simulink model "svpwm"  (R2021b)
settings: Solver=FixedStepDiscrete  StartTime=0.0  StopTime=0.5  FixedStep=sysStep  RelTol=1e-3
InitFcn:
  | % 华为参数
  | sysStep = 0.5e-6;
  | Udc = 300;
  | PrdPwmCarr = 3125;
  | Ts = 2e-8 * PrdPwmCarr;
  | en7SecMod = true;
  | enModulationUp = true;
  | deadtimeDelay = uint8(5e-6/sysStep); %5us deadtime
  | 
  | %电机参数
  | polepairs = 4;
libraries: spsDiodeLib x6, spsIGBTLib x6, spsVoltageMeasurementLib x3, spsDCVoltageSourceLib x2, spsParallelRLCBranchLib x2, spsGroundLib x1, spsPermanentMagnetSynchronousMachineLib x1, spspowerguiLib x1, simulink x1
settings Model: Creator=zqzq_  LastModifiedBy=zqzq_

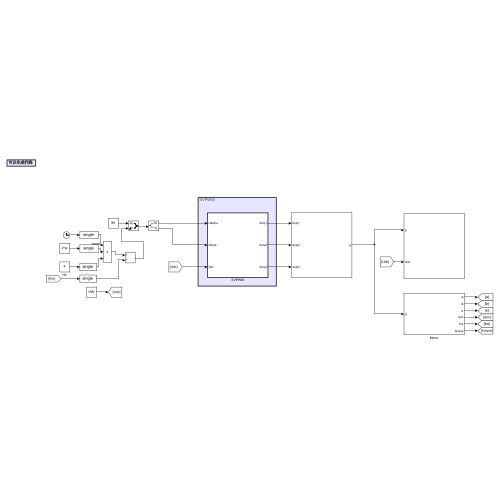
[thumbnail: Simulink's stored preview of the top-level diagram]
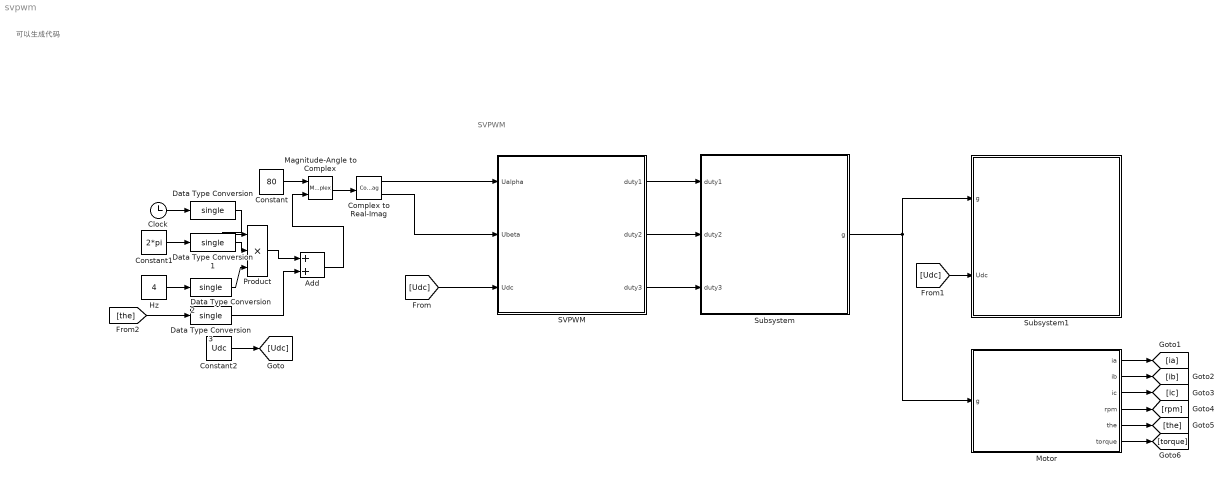
== system svpwm ==
  note: 可以生成代码
  note: SVPWM
  Add : Sum
  Clock : Clock
  Complex to Real-Imag : ComplexToRealImag
  Constant : Constant  Value=80  OutDataTypeStr=Inherit: Inherit via back propagation
  Constant1 : Constant  Value=2*pi  OutDataTypeStr=Inherit: Inherit via back propagation
  Constant2 : Constant  Value=Udc  OutDataTypeStr=Inherit: Inherit via back propagation
  Data Type Conversion{,1..3} (4 alike) : DataTypeConversion  OutDataTypeStr=single
  Hz : Constant  Value=4  OutDataTypeStr=Inherit: Inherit via back propagation
  Magnitude-Angle to Complex : MagnitudeAngleToComplex
  Motor : Subsystem
  Product : Product  Inputs=3
  SVPWM : Subsystem  TreatAsAtomicUnit=on
  Subsystem : Subsystem
  Subsystem1 : Subsystem
  wires:
  Constant2/1 -> [Udc]
  Constant/1 -> Magnitude-Angle to Complex/1
  Complex to Real-Imag/1 -> SVPWM/1(Ualpha)
  Complex to Real-Imag/2 -> SVPWM/2(Ubeta)
  Magnitude-Angle to Complex/1 -> Complex to Real-Imag/1
  Clock/1 -> Data Type Conversion/1
  Constant1/1 -> Data Type Conversion1/1
  Hz/1 -> Data Type Conversion2/1
  Add/1 -> Magnitude-Angle to Complex/2
  Data Type Conversion/1 -> Product/1
  Data Type Conversion1/1 -> Product/2
  Data Type Conversion2/1 -> Product/3
  SVPWM/1(duty1) -> Subsystem/1(duty1)
  SVPWM/2(duty2) -> Subsystem/2(duty2)
  SVPWM/3(duty3) -> Subsystem/3(duty3)
  Subsystem/1(g) -> Motor/1(g), Subsystem1/1(g)
  [Udc] -> SVPWM/3(Udc)
  [Udc] -> Subsystem1/2(Udc)
  Motor/1(ia) -> [ia]
  Motor/2(ib) -> [ib]
  Motor/3(ic) -> [ic]
  Motor/4(rpm) -> [rpm]
  Motor/5(the) -> [the]
  Motor/6(torque) -> [torque]
  [the] -> Data Type Conversion3/1
  Product/1 -> Add/1
  Data Type Conversion3/1 -> Add/2

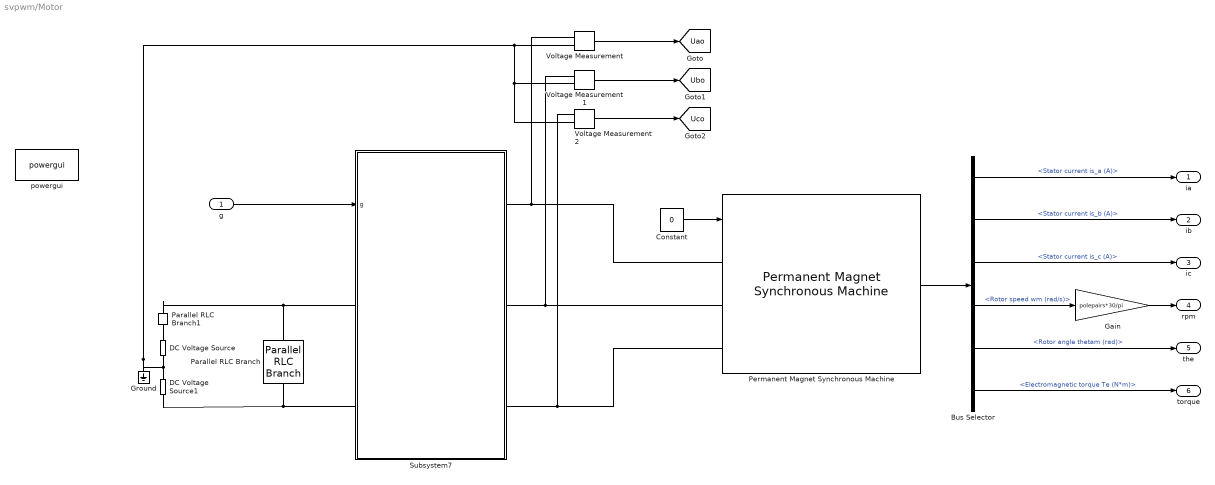
== system svpwm/Motor ==
  g : Inport
  Bus Selector : BusSelector  OutputSignals=Stator current is_a (A),Stator current is_b (A),Stator current is_c (A),Rotor speed wm (rad/s),Rotor angle thetam (rad),Electromagnetic torque Te (N*m)
  Constant : Constant  Value=0  OutDataTypeStr=Inherit: Inherit via back propagation
  DC Voltage Source : spsDCVoltageSourceLib/DC Voltage Source  Amplitude=Udc/2  Measurements=None
  DC Voltage Source1 : spsDCVoltageSourceLib/DC Voltage Source  Amplitude=Udc/2  Measurements=None
  Gain : Gain  Gain=polepairs*30/pi
  Ground : spsGroundLib/Ground  LConnTagsString=a
  Parallel RLC Branch : spsParallelRLCBranchLib/Parallel RLC Branch  LConnTagsString=a  RConnTagsString=__new0  BranchType=C  Resistance=1  Inductance=1e-3  SetiL0=off  InitialCurrent=0  Capacitance=50e-6  Setx0=on  InitialVoltage=Udc  Measurements=None
  Parallel RLC Branch1 : spsParallelRLCBranchLib/Parallel RLC Branch  LConnTagsString=a  RConnTagsString=__new0  BranchType=R  Resistance=0.01  Inductance=1e-3  SetiL0=off  InitialCurrent=0  Capacitance=50e-6  Setx0=on  InitialVoltage=Udc  Measurements=None
  Permanent Magnet Synchronous Machine : spsPermanentMagnetSynchronousMachineLib/Permanent Magnet Synchronous Machine  NbPhases=3  FluxDistribution=Sinusoidal  RotorType=Salient-pole  MechanicalLoad=Speed w  PresetModel="10:  7.71 Nm 560 Vdc 5000 RPM - 10.2 Nm"  ShowDetailedParameters=on  MeasurementBus=off  Resistance=0.18  Inductance=8.5e-3  dqInductances=[0.0007932 0.0008767]  La=0.00097  MachineConstant=Flux linkage established by magnets (V.s)  Flux=0.07145  VoltageCst=51.8384  TorqueCst=0.4287  Flat=120  Mechanical=[0.00062 0.0003035 4 0]  PolePairs=4  InitialConditions=[0,0, 0,0]  InitialConditions5ph=[0 0 0 0 0 0]  RefAngle=90 degrees behind phase A axis (modified Park)  IterativeDiscreteModel=Trapezoidal non iterative  TsBlock=-1  TsPowergui=0
  Subsystem7 : Subsystem
  Voltage Measurement : spsVoltageMeasurementLib/Voltage Measurement  PhasorSimulation=off  OutputType=Complex  PSBequivalent=0
  Voltage Measurement1 : spsVoltageMeasurementLib/Voltage Measurement  PhasorSimulation=off  OutputType=Complex  PSBequivalent=0
  Voltage Measurement2 : spsVoltageMeasurementLib/Voltage Measurement  PhasorSimulation=off  OutputType=Complex  PSBequivalent=0
  powergui : spspowerguiLib/powergui  Priority=1  SimulationMode=Discrete  SampleTime=sysStep  frequency=60  Iterations=50  frequencyindice=0  Pbase=100e6  ErrMax=1e-4  UnitsV=kV  UnitsW=MW  buscounter=0  FunctionMessages=off  echomessages=off  EnableUseOfTLC=off  CurrentSourceSwitches=off  DisableSnubberDevices=off  DisableRonSwitches=off  DisableVfSwitches=off  DisplayEquations=off  AutomaticDiscreteSolvers=off  SolverType=Tustin/Backward Euler (TBE)  Interpol=off  ExternalGateDelay=off  methode=off  Ts=100  x0status=blocks  SPID=on  SwTol=0  HookPort=off  NonlinearTolerance=1e-4  nMaxIteration=100  ContinueOnMaxIteration=off  RestoreLinks=warning  ResistiveCurrentMeasurement=off  Frange=[0:2:500]  Ylog=off  Xlog=on  ShowGrid=off  save=off  variable=ZData  structure=0  ZoomFFT=off  StartTime=0.0  cycles=1  DisplayStyle=1  fundamental=60  FreqAxis=off  MaxFrequency=1000  frequencyindicesteady=1  RmsSteady=1  display=off
  ia : Outport
  ib : Outport  Port=2
  ic : Outport  Port=3
  rpm : Outport  Port=4
  the : Outport  Port=5
  torque : Outport  Port=6
  tag scope: Uao=global, Ubo=global, Uco=global
  wires:
  g/1 -> Subsystem7/1(g)
  Permanent Magnet Synchronous Machine/1 -> Bus Selector/1
  Voltage Measurement/1 -> [Uao]
  Voltage Measurement1/1 -> [Ubo]
  Voltage Measurement2/1 -> [Uco]
  Bus Selector/1 -> ia/1  "<Stator current is_a (A)>"
  Bus Selector/2 -> ib/1  "<Stator current is_b (A)>"
  Bus Selector/3 -> ic/1  "<Stator current is_c (A)>"
  Bus Selector/4 -> Gain/1  "<Rotor speed wm (rad/s)>"
  Bus Selector/5 -> the/1  "<Rotor angle thetam (rad)>"
  Bus Selector/6 -> torque/1  "<Electromagnetic torque Te (N*m)>"
  Gain/1 -> rpm/1
  Constant/1 -> Permanent Magnet Synchronous Machine/1
  connections:
  Subsystem7/RConn2 -- Voltage Measurement1/LConn1 -- Permanent Magnet Synchronous Machine/LConn2
  Parallel RLC Branch/LConn1 -- Parallel RLC Branch1/LConn1 -- Subsystem7/LConn1
  Subsystem7/RConn3 -- Voltage Measurement2/LConn1 -- Permanent Magnet Synchronous Machine/LConn3
  Subsystem7/RConn1 -- Voltage Measurement/LConn1 -- Permanent Magnet Synchronous Machine/LConn1
  Parallel RLC Branch/RConn1 -- DC Voltage Source1/LConn1 -- Subsystem7/LConn2
  Parallel RLC Branch1/RConn1 -- DC Voltage Source/RConn1
  DC Voltage Source/LConn1 -- Voltage Measurement2/LConn2 -- Voltage Measurement1/LConn2 -- Voltage Measurement/LConn2 -- Ground/LConn1 -- DC Voltage Source1/RConn1

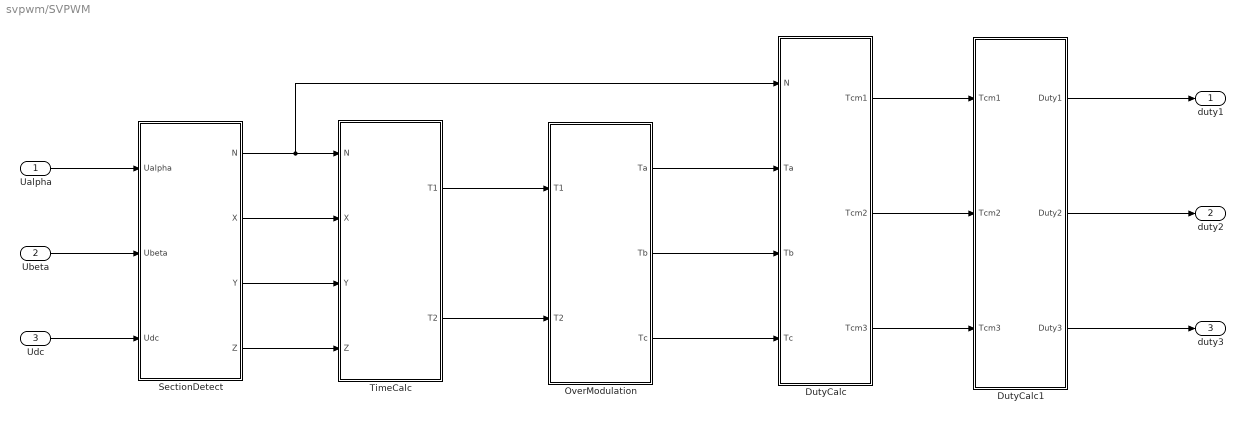
== system svpwm/SVPWM ==
  Ualpha : Inport
  Ubeta : Inport  Port=2
  Udc : Inport  Port=3
  DutyCalc : Subsystem  TreatAsAtomicUnit=on
  DutyCalc1 : Subsystem  TreatAsAtomicUnit=on
  OverModulation : Subsystem  TreatAsAtomicUnit=on
  SectionDetect : Subsystem  TreatAsAtomicUnit=on
  TimeCalc : Subsystem  TreatAsAtomicUnit=on
  duty1 : Outport
  duty2 : Outport  Port=2
  duty3 : Outport  Port=3
  wires:
  Ualpha/1 -> SectionDetect/1(Ualpha)
  Ubeta/1 -> SectionDetect/2(Ubeta)
  Udc/1 -> SectionDetect/3(Udc)
  SectionDetect/1(N) -> DutyCalc/1(N), TimeCalc/1(N)
  SectionDetect/2(X) -> TimeCalc/2(X)
  SectionDetect/3(Y) -> TimeCalc/3(Y)
  SectionDetect/4(Z) -> TimeCalc/4(Z)
  TimeCalc/1(T1) -> OverModulation/1(T1)
  TimeCalc/2(T2) -> OverModulation/2(T2)
  OverModulation/1(Ta) -> DutyCalc/2(Ta)
  OverModulation/2(Tb) -> DutyCalc/3(Tb)
  OverModulation/3(Tc) -> DutyCalc/4(Tc)
  DutyCalc/1(Tcm1) -> DutyCalc1/1(Tcm1)
  DutyCalc/2(Tcm2) -> DutyCalc1/2(Tcm2)
  DutyCalc/3(Tcm3) -> DutyCalc1/3(Tcm3)
  DutyCalc1/1(Duty1) -> duty1/1
  DutyCalc1/3(Duty3) -> duty3/1
  DutyCalc1/2(Duty2) -> duty2/1

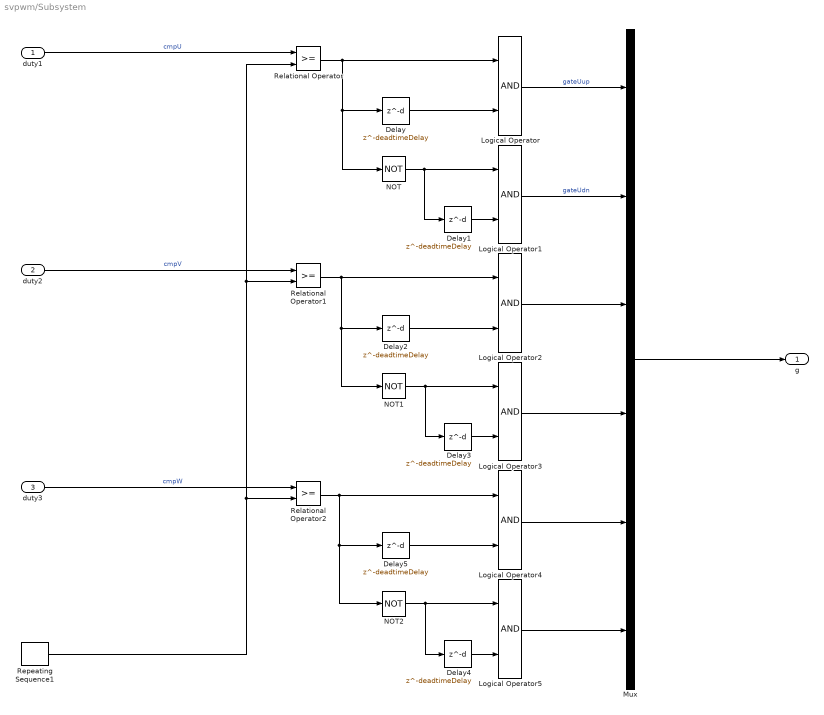
== system svpwm/Subsystem ==
  duty1 : Inport
  duty2 : Inport  Port=2
  duty3 : Inport  Port=3
  Delay{,1..5} (6 alike) : Delay  DelayLength=deadtimeDelay
  Logical Operator{,1..5} (6 alike) : Logic  AllPortsSameDT=off  OutDataTypeStr=boolean
  Mux : Mux  Inputs=6
  NOT : Logic  Operator=NOT  AllPortsSameDT=off  OutDataTypeStr=boolean
  NOT1 : Logic  Operator=NOT  AllPortsSameDT=off  OutDataTypeStr=boolean
  NOT2 : Logic  Operator=NOT  AllPortsSameDT=off  OutDataTypeStr=boolean
  Relational Operator : RelationalOperator  OutDataTypeStr=boolean  RndMeth=Simplest
  Relational Operator1 : RelationalOperator  OutDataTypeStr=boolean  RndMeth=Simplest
  Relational Operator2 : RelationalOperator  OutDataTypeStr=boolean  RndMeth=Simplest
  Repeating Sequence1 : simulink/Sources/Repeating Sequence  rep_seq_t=[0 2e-8*PrdPwmCarr 4e-8*PrdPwmCarr]  rep_seq_y=[0.001 0.999 0.001]
  g : Outport
  wires:
  duty1/1 -> Relational Operator/1  "cmpU"
  duty2/1 -> Relational Operator1/1  "cmpV"
  Mux/1 -> g/1
  Logical Operator/1 -> Mux/1  "gateUup"
  Logical Operator1/1 -> Mux/2  "gateUdn"
  Logical Operator2/1 -> Mux/3
  Logical Operator3/1 -> Mux/4
  Logical Operator4/1 -> Mux/5
  Logical Operator5/1 -> Mux/6
  Repeating Sequence1/1 -> Relational Operator2/2, Relational Operator/2, Relational Operator1/2
  Relational Operator/1 -> Delay/1, NOT/1, Logical Operator/1
  NOT/1 -> Delay1/1, Logical Operator1/1
  duty3/1 -> Relational Operator2/1  "cmpW"
  NOT1/1 -> Delay3/1, Logical Operator3/1
  Relational Operator1/1 -> Delay2/1, NOT1/1, Logical Operator2/1
  NOT2/1 -> Delay4/1, Logical Operator5/1
  Delay/1 -> Logical Operator/2
  Delay1/1 -> Logical Operator1/2
  Delay2/1 -> Logical Operator2/2
  Delay3/1 -> Logical Operator3/2
  Delay4/1 -> Logical Operator5/2
  Relational Operator2/1 -> Delay5/1, NOT2/1, Logical Operator4/1
  Delay5/1 -> Logical Operator4/2

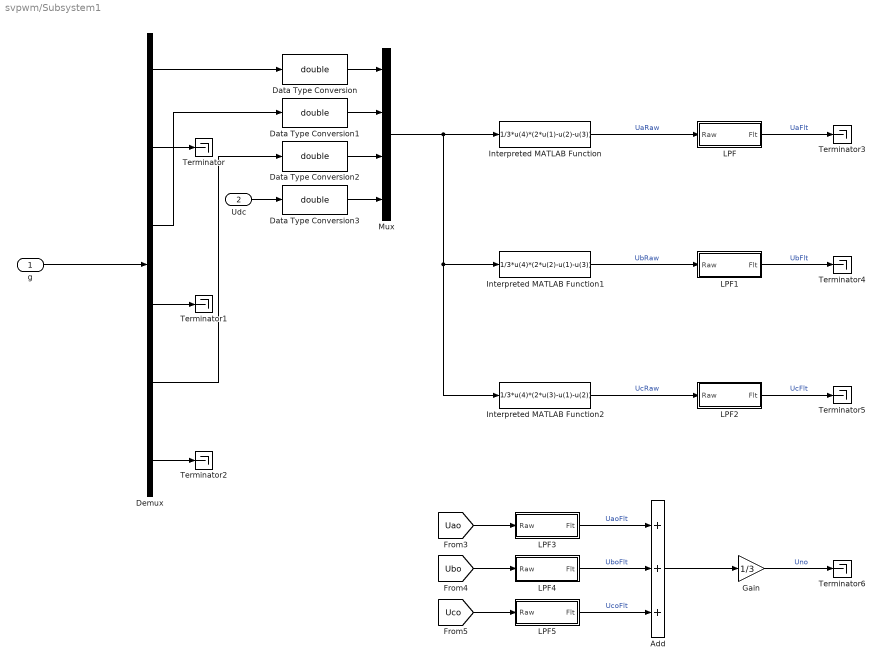
== system svpwm/Subsystem1 ==
  g : Inport
  Udc : Inport  Port=2  OutDataTypeStr=single
  Add : Sum  Inputs=+++
  Data Type Conversion{,1..3} (4 alike) : DataTypeConversion  OutDataTypeStr=double
  Demux : Demux  Outputs=6
  Gain : Gain  Gain=1/3
  Interpreted MATLAB Function : MATLABFcn  MATLABFcn=1/3*u(4)*(2*u(1)-u(2)-u(3))  OutputSignalType=real
  Interpreted MATLAB Function1 : MATLABFcn  MATLABFcn=1/3*u(4)*(2*u(2)-u(1)-u(3))  OutputSignalType=real
  Interpreted MATLAB Function2 : MATLABFcn  MATLABFcn=1/3*u(4)*(2*u(3)-u(1)-u(2))  OutputSignalType=real
  LPF : Subsystem  TreatAsAtomicUnit=on
  LPF1 : Subsystem  TreatAsAtomicUnit=on
  LPF2 : Subsystem  TreatAsAtomicUnit=on
  LPF3 : Subsystem  TreatAsAtomicUnit=on
  LPF4 : Subsystem  TreatAsAtomicUnit=on
  LPF5 : Subsystem  TreatAsAtomicUnit=on
  Mux : Mux
  Terminator{,1..6} (7 alike) : Terminator
  wires:
  g/1 -> Demux/1
  Demux/2 -> Terminator/1
  Demux/4 -> Terminator1/1
  Demux/6 -> Terminator2/1
  Demux/1 -> Data Type Conversion/1
  Demux/3 -> Data Type Conversion1/1
  Demux/5 -> Data Type Conversion2/1
  Udc/1 -> Data Type Conversion3/1
  Interpreted MATLAB Function/1 -> LPF/1(Raw)  "UaRaw"
  Interpreted MATLAB Function1/1 -> LPF1/1(Raw)  "UbRaw"
  Interpreted MATLAB Function2/1 -> LPF2/1(Raw)  "UcRaw"
  Mux/1 -> Interpreted MATLAB Function2/1, Interpreted MATLAB Function1/1, Interpreted MATLAB Function/1
  Data Type Conversion/1 -> Mux/1
  Data Type Conversion1/1 -> Mux/2
  Data Type Conversion2/1 -> Mux/3
  Data Type Conversion3/1 -> Mux/4
  LPF/1(Flt) -> Terminator3/1  "UaFlt"
  LPF1/1(Flt) -> Terminator4/1  "UbFlt"
  LPF2/1(Flt) -> Terminator5/1  "UcFlt"
  Add/1 -> Gain/1
  Gain/1 -> Terminator6/1  "Uno"
  [Uao] -> LPF3/1(Raw)
  [Ubo] -> LPF4/1(Raw)
  [Uco] -> LPF5/1(Raw)
  LPF3/1(Flt) -> Add/1  "UaoFlt"
  LPF4/1(Flt) -> Add/2  "UboFlt"
  LPF5/1(Flt) -> Add/3  "UcoFlt"

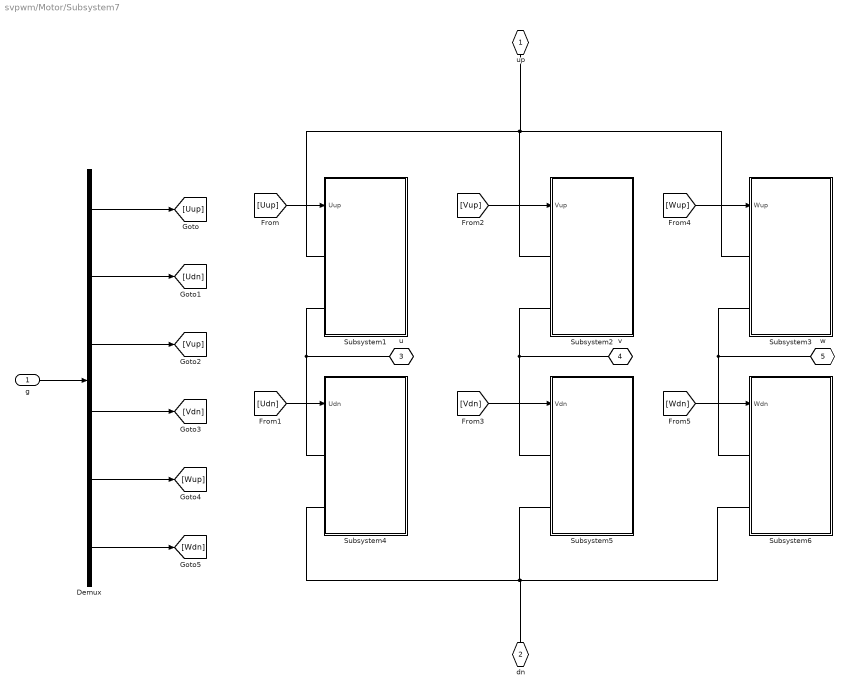
== system svpwm/Motor/Subsystem7 ==
  g : Inport
  Demux : Demux  Outputs=6
  Subsystem1 : Subsystem
  Subsystem2 : Subsystem
  Subsystem3 : Subsystem
  Subsystem4 : Subsystem
  Subsystem5 : Subsystem
  Subsystem6 : Subsystem
  up : PMIOPort  Side=Left
  dn : PMIOPort  Port=2  Side=Left
  u : PMIOPort  Port=3  Side=Right
  v : PMIOPort  Port=4  Side=Right
  w : PMIOPort  Port=5  Side=Right
  wires:
  g/1 -> Demux/1
  Demux/1 -> [Uup]
  Demux/2 -> [Udn]
  Demux/3 -> [Vup]
  Demux/4 -> [Vdn]
  Demux/5 -> [Wup]
  Demux/6 -> [Wdn]
  [Uup] -> Subsystem1/1(Uup)
  [Udn] -> Subsystem4/1(Udn)
  [Vup] -> Subsystem2/1(Vup)
  [Vdn] -> Subsystem5/1(Vdn)
  [Wup] -> Subsystem3/1(Wup)
  [Wdn] -> Subsystem6/1(Wdn)
  connections:
  Subsystem3/LConn2 -- w/RConn1 -- Subsystem6/LConn1
  Subsystem4/LConn2 -- Subsystem6/LConn2 -- dn/RConn1 -- Subsystem5/LConn2
  Subsystem1/LConn1 -- Subsystem3/LConn1 -- up/RConn1 -- Subsystem2/LConn1
  Subsystem2/LConn2 -- v/RConn1 -- Subsystem5/LConn1
  Subsystem1/LConn2 -- u/RConn1 -- Subsystem4/LConn1

== system svpwm/SVPWM/DutyCalc ==
  N : Inport
  Ta : Inport  Port=2
  Tb : Inport  Port=3
  Tc : Inport  Port=4
  Multiport Switch : MultiPortSwitch  Inputs=6
  Multiport Switch1 : MultiPortSwitch  Inputs=6
  Multiport Switch2 : MultiPortSwitch  Inputs=6
  Tcm1 : Outport
  Tcm2 : Outport  Port=2
  Tcm3 : Outport  Port=3
  wires:
  Multiport Switch2/1 -> Tcm3/1
  Multiport Switch1/1 -> Tcm2/1
  Multiport Switch/1 -> Tcm1/1
  Ta/1 -> Multiport Switch2/7, Multiport Switch2/5, Multiport Switch1/6, Multiport Switch1/2, Multiport Switch/3, Multiport Switch/4
  Tb/1 -> Multiport Switch2/6, Multiport Switch2/3, Multiport Switch1/5, Multiport Switch1/4, Multiport Switch/7, Multiport Switch/2
  N/1 -> Multiport Switch2/1, Multiport Switch1/1, Multiport Switch/1
  Tc/1 -> Multiport Switch2/4, Multiport Switch/6, Multiport Switch/5, Multiport Switch1/3, Multiport Switch1/7, Multiport Switch2/2

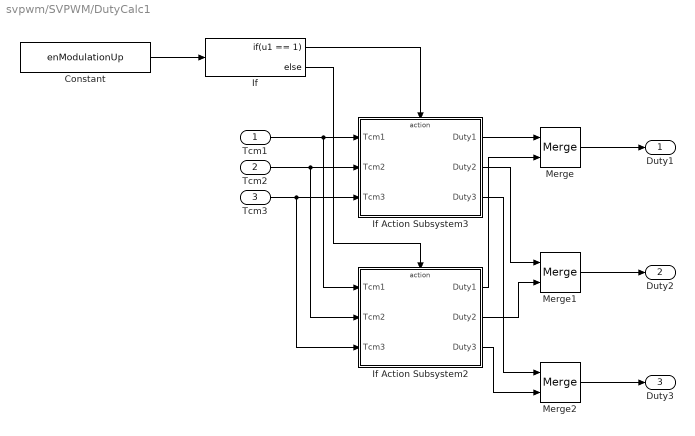
== system svpwm/SVPWM/DutyCalc1 ==
  Tcm1 : Inport
  Tcm2 : Inport  Port=2
  Tcm3 : Inport  Port=3
  Constant : Constant  Value=enModulationUp
  If : If  IfExpression=u1 == 1
  If Action Subsystem2 : Subsystem  TreatAsAtomicUnit=on
  If Action Subsystem3 : Subsystem  TreatAsAtomicUnit=on
  Merge : Merge
  Merge1 : Merge
  Merge2 : Merge
  Duty1 : Outport
  Duty2 : Outport  Port=2
  Duty3 : Outport  Port=3
  wires:
  Constant/1 -> If/1
  If/1 -> If Action Subsystem3/Action
  Tcm1/1 -> If Action Subsystem2/1(Tcm1), If Action Subsystem3/1(Tcm1)
  Tcm2/1 -> If Action Subsystem2/2(Tcm2), If Action Subsystem3/2(Tcm2)
  Tcm3/1 -> If Action Subsystem2/3(Tcm3), If Action Subsystem3/3(Tcm3)
  If Action Subsystem3/1(Duty1) -> Merge/1
  If/2 -> If Action Subsystem2/Action
  Merge/1 -> Duty1/1
  Merge1/1 -> Duty2/1
  If Action Subsystem3/2(Duty2) -> Merge1/1
  Merge2/1 -> Duty3/1
  If Action Subsystem3/3(Duty3) -> Merge2/1
  If Action Subsystem2/3(Duty3) -> Merge2/2
  If Action Subsystem2/2(Duty2) -> Merge1/2
  If Action Subsystem2/1(Duty1) -> Merge/2

== system svpwm/SVPWM/OverModulation ==
  T1 : Inport
  T2 : Inport  Port=2
  OverModulationCalc : Subsystem  TreatAsAtomicUnit=on
  TabcCalc : Subsystem  TreatAsAtomicUnit=on
  Ta : Outport
  Tb : Outport  Port=2
  Tc : Outport  Port=3
  wires:
  T2/1 -> OverModulationCalc/2(T2)
  T1/1 -> OverModulationCalc/1(T1)
  OverModulationCalc/2(T2_) -> TabcCalc/2(T2_)
  TabcCalc/1(Ta) -> Ta/1
  TabcCalc/2(Tb) -> Tb/1
  TabcCalc/3(Tc) -> Tc/1
  OverModulationCalc/1(T1_) -> TabcCalc/1(T1_)

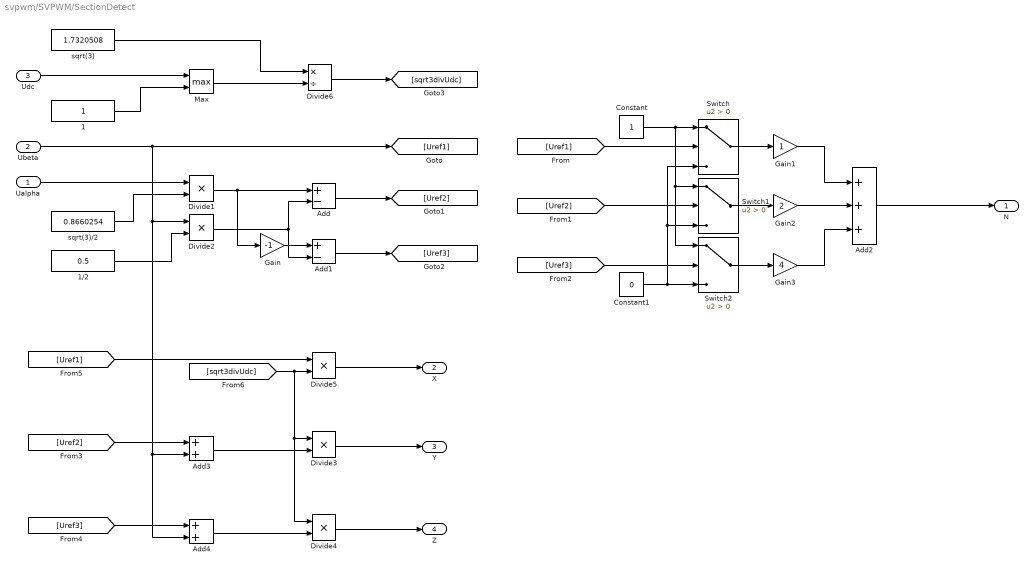
== system svpwm/SVPWM/SectionDetect ==
  Ualpha : Inport
  Ubeta : Inport  Port=2
  Udc : Inport  Port=3
  1 : Constant  OutDataTypeStr=single
  1/2 : Constant  Value=0.5  OutDataTypeStr=single
  Add : Sum  Inputs=+-
  Add1 : Sum  Inputs=+-
  Add2 : Sum  Inputs=+++
  Add3 : Sum
  Add4 : Sum
  Constant : Constant  OutDataTypeStr=uint8
  Constant1 : Constant  Value=0  OutDataTypeStr=uint8
  Divide{1..5} (5 alike) : Product  Inputs=**
  Divide6 : Product  Inputs=*/
  Gain : Gain  Gain=-1
  Gain1 : Gain
  Gain2 : Gain  Gain=2
  Gain3 : Gain  Gain=4
  Max : MinMax  Function=max  Inputs=2
  Switch : Switch  Criteria=u2 > Threshold
  Switch1 : Switch  Criteria=u2 > Threshold
  Switch2 : Switch  Criteria=u2 > Threshold
  sqrt(3) : Constant  Value=1.7320508  OutDataTypeStr=single
  sqrt(3)/2 : Constant  Value=0.8660254  OutDataTypeStr=single
  N : Outport
  X : Outport  Port=2
  Y : Outport  Port=3
  Z : Outport  Port=4
  wires:
  Ubeta/1 -> [Uref1], Add4/2, Add3/2, Divide2/1
  Ualpha/1 -> Divide1/1
  Divide1/1 -> Gain/1, Add/1
  sqrt(3)/2/1 -> Divide1/2
  1/2/1 -> Divide2/2
  Add/1 -> [Uref2]
  Divide2/1 -> Add1/2, Add/2
  Add1/1 -> [Uref3]
  Gain/1 -> Add1/1
  [Uref1] -> Switch/2
  Constant/1 -> Switch2/1, Switch1/1, Switch/1
  Constant1/1 -> Switch/3, Switch1/3, Switch2/3
  Switch/1 -> Gain1/1
  [Uref2] -> Switch1/2
  Switch1/1 -> Gain2/1
  Switch2/1 -> Gain3/1
  [Uref3] -> Switch2/2
  Gain2/1 -> Add2/2
  Gain1/1 -> Add2/1
  Gain3/1 -> Add2/3
  Add2/1 -> N/1
  [Uref2] -> Add3/1
  [Uref3] -> Add4/1
  Add3/1 -> Divide3/2
  Add4/1 -> Divide4/2
  [Uref1] -> Divide5/1
  Udc/1 -> Max/1
  1/1 -> Max/2
  Max/1 -> Divide6/2
  sqrt(3)/1 -> Divide6/1
  Divide6/1 -> [sqrt3divUdc]
  [sqrt3divUdc] -> Divide3/1, Divide4/1, Divide5/2
  Divide5/1 -> X/1
  Divide3/1 -> Y/1
  Divide4/1 -> Z/1

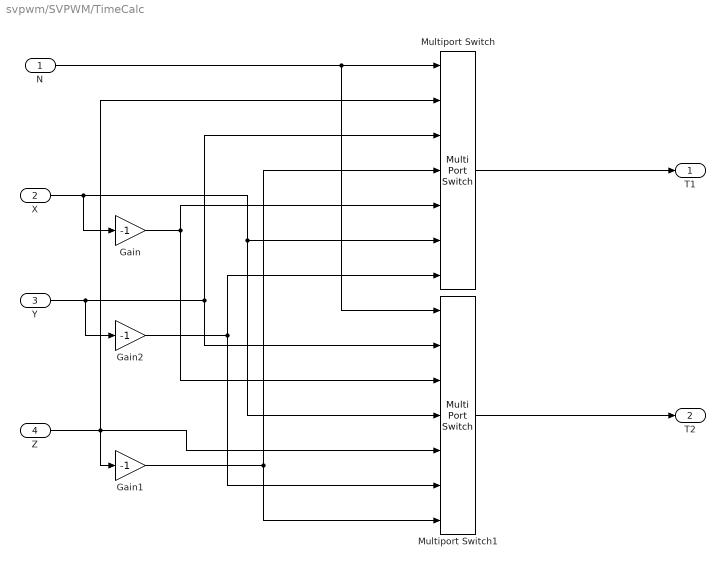
== system svpwm/SVPWM/TimeCalc ==
  N : Inport
  X : Inport  Port=2
  Y : Inport  Port=3
  Z : Inport  Port=4
  Gain : Gain  Gain=-1
  Gain1 : Gain  Gain=-1
  Gain2 : Gain  Gain=-1
  Multiport Switch : MultiPortSwitch  Inputs=6
  Multiport Switch1 : MultiPortSwitch  Inputs=6
  T1 : Outport
  T2 : Outport  Port=2
  wires:
  N/1 -> Multiport Switch1/1, Multiport Switch/1
  Z/1 -> Multiport Switch1/5, Gain1/1, Multiport Switch/2
  X/1 -> Multiport Switch1/4, Multiport Switch/6, Gain/1
  Gain/1 -> Multiport Switch/5, Multiport Switch1/3
  Y/1 -> Multiport Switch/3, Multiport Switch1/2, Gain2/1
  Gain2/1 -> Multiport Switch1/6, Multiport Switch/7
  Gain1/1 -> Multiport Switch/4, Multiport Switch1/7
  Multiport Switch/1 -> T1/1
  Multiport Switch1/1 -> T2/1

== system svpwm/Subsystem1/LPF ==
  Raw : Inport
  Add : Sum
  Add1 : Sum  Inputs=+-
  Constant : Constant  Value=0.001  OutDataTypeStr=Inherit: Inherit via back propagation
  Constant1 : Constant  OutDataTypeStr=Inherit: Inherit via back propagation
  Delay : Delay  DelayLength=1
  Product : Product
  Product1 : Product
  Flt : Outport
  wires:
  Raw/1 -> Product1/1
  Add/1 -> Delay/1, Flt/1
  Delay/1 -> Product/2
  Product/1 -> Add/2
  Constant/1 -> Add1/2, Product1/2
  Product1/1 -> Add/1
  Add1/1 -> Product/1
  Constant1/1 -> Add1/1

== system svpwm/Subsystem1/LPF1 ==
  Raw : Inport
  Add : Sum
  Add1 : Sum  Inputs=+-
  Constant : Constant  Value=0.001  OutDataTypeStr=Inherit: Inherit via back propagation
  Constant1 : Constant  OutDataTypeStr=Inherit: Inherit via back propagation
  Delay : Delay  DelayLength=1
  Product : Product
  Product1 : Product
  Flt : Outport
  wires:
  Constant1/1 -> Add1/1
  Add1/1 -> Product/1
  Product1/1 -> Add/1
  Constant/1 -> Product1/2, Add1/2
  Product/1 -> Add/2
  Delay/1 -> Product/2
  Add/1 -> Flt/1, Delay/1
  Raw/1 -> Product1/1

== system svpwm/Subsystem1/LPF2 ==
  Raw : Inport
  Add : Sum
  Add1 : Sum  Inputs=+-
  Constant : Constant  Value=0.001  OutDataTypeStr=Inherit: Inherit via back propagation
  Constant1 : Constant  OutDataTypeStr=Inherit: Inherit via back propagation
  Delay : Delay  DelayLength=1
  Product : Product
  Product1 : Product
  Flt : Outport
  wires:
  Raw/1 -> Product1/1
  Add/1 -> Delay/1, Flt/1
  Delay/1 -> Product/2
  Product/1 -> Add/2
  Constant/1 -> Add1/2, Product1/2
  Product1/1 -> Add/1
  Add1/1 -> Product/1
  Constant1/1 -> Add1/1

== system svpwm/Subsystem1/LPF3 ==
  Raw : Inport
  Add : Sum
  Add1 : Sum  Inputs=+-
  Constant : Constant  Value=0.0004  OutDataTypeStr=Inherit: Inherit via back propagation
  Constant1 : Constant  OutDataTypeStr=Inherit: Inherit via back propagation
  Delay : Delay  DelayLength=1
  Product : Product
  Product1 : Product
  Flt : Outport
  wires:
  Constant1/1 -> Add1/1
  Add1/1 -> Product/1
  Product1/1 -> Add/1
  Constant/1 -> Product1/2, Add1/2
  Product/1 -> Add/2
  Delay/1 -> Product/2
  Add/1 -> Flt/1, Delay/1
  Raw/1 -> Product1/1

== system svpwm/Subsystem1/LPF4 ==
  Raw : Inport
  Add : Sum
  Add1 : Sum  Inputs=+-
  Constant : Constant  Value=0.0004  OutDataTypeStr=Inherit: Inherit via back propagation
  Constant1 : Constant  OutDataTypeStr=Inherit: Inherit via back propagation
  Delay : Delay  DelayLength=1
  Product : Product
  Product1 : Product
  Flt : Outport
  wires:
  Raw/1 -> Product1/1
  Add/1 -> Delay/1, Flt/1
  Delay/1 -> Product/2
  Product/1 -> Add/2
  Constant/1 -> Add1/2, Product1/2
  Product1/1 -> Add/1
  Add1/1 -> Product/1
  Constant1/1 -> Add1/1

== system svpwm/Subsystem1/LPF5 ==
  Raw : Inport
  Add : Sum
  Add1 : Sum  Inputs=+-
  Constant : Constant  Value=0.0004  OutDataTypeStr=Inherit: Inherit via back propagation
  Constant1 : Constant  OutDataTypeStr=Inherit: Inherit via back propagation
  Delay : Delay  DelayLength=1
  Product : Product
  Product1 : Product
  Flt : Outport
  wires:
  Constant1/1 -> Add1/1
  Add1/1 -> Product/1
  Product1/1 -> Add/1
  Constant/1 -> Product1/2, Add1/2
  Product/1 -> Add/2
  Delay/1 -> Product/2
  Add/1 -> Flt/1, Delay/1
  Raw/1 -> Product1/1

== system svpwm/Motor/Subsystem7/Subsystem1 ==
  Uup : Inport
  Diode : spsDiodeLib/Diode  Ron=0.001  Lon=0  Vf=0.8  IC=0  UseSnubber=0  Rs=500  Cs=250e-9  Measurements=on
  IGBT : spsIGBTLib/IGBT  Ron=0.001  Lon=0  Vf=1  Tf=1e-6  Tt=2e-6  IC=0  Rs=1e5  Cs=inf  Measurements=on
  Terminator : Terminator
  Terminator1 : Terminator
  up : PMIOPort  Side=Left
  dn : PMIOPort  Port=2  Side=Left
  wires:
  Diode/1 -> Terminator/1
  IGBT/1 -> Terminator1/1
  Uup/1 -> IGBT/1
  connections:
  Diode/LConn1 -- dn/RConn1 -- IGBT/RConn1
  Diode/RConn1 -- IGBT/LConn1 -- up/RConn1

== system svpwm/Motor/Subsystem7/Subsystem2 ==
  Vup : Inport
  Diode : spsDiodeLib/Diode  Ron=0.001  Lon=0  Vf=0.8  IC=0  UseSnubber=0  Rs=500  Cs=250e-9  Measurements=on
  IGBT : spsIGBTLib/IGBT  Ron=0.001  Lon=0  Vf=1  Tf=1e-6  Tt=2e-6  IC=0  Rs=1e5  Cs=inf  Measurements=on
  Terminator : Terminator
  Terminator1 : Terminator
  up : PMIOPort  Side=Left
  dn : PMIOPort  Port=2  Side=Left
  wires:
  Vup/1 -> IGBT/1
  IGBT/1 -> Terminator1/1
  Diode/1 -> Terminator/1
  connections:
  IGBT/LConn1 -- Diode/RConn1 -- up/RConn1
  dn/RConn1 -- Diode/LConn1 -- IGBT/RConn1

== system svpwm/Motor/Subsystem7/Subsystem3 ==
  Wup : Inport
  Diode : spsDiodeLib/Diode  Ron=0.001  Lon=0  Vf=0.8  IC=0  UseSnubber=0  Rs=500  Cs=250e-9  Measurements=on
  IGBT : spsIGBTLib/IGBT  Ron=0.001  Lon=0  Vf=1  Tf=1e-6  Tt=2e-6  IC=0  Rs=1e5  Cs=inf  Measurements=on
  Terminator : Terminator
  Terminator1 : Terminator
  up : PMIOPort  Side=Left
  dn : PMIOPort  Port=2  Side=Left
  wires:
  Diode/1 -> Terminator/1
  IGBT/1 -> Terminator1/1
  Wup/1 -> IGBT/1
  connections:
  IGBT/RConn1 -- Diode/LConn1 -- dn/RConn1
  up/RConn1 -- Diode/RConn1 -- IGBT/LConn1

== system svpwm/Motor/Subsystem7/Subsystem4 ==
  Udn : Inport
  Diode : spsDiodeLib/Diode  Ron=0.001  Lon=0  Vf=0.8  IC=0  UseSnubber=0  Rs=500  Cs=250e-9  Measurements=on
  IGBT : spsIGBTLib/IGBT  Ron=0.001  Lon=0  Vf=1  Tf=1e-6  Tt=2e-6  IC=0  Rs=1e5  Cs=inf  Measurements=on
  Terminator : Terminator
  Terminator1 : Terminator
  up : PMIOPort  Side=Left
  dn : PMIOPort  Port=2  Side=Left
  wires:
  Udn/1 -> IGBT/1
  IGBT/1 -> Terminator1/1
  Diode/1 -> Terminator/1
  connections:
  IGBT/LConn1 -- Diode/RConn1 -- up/RConn1
  dn/RConn1 -- Diode/LConn1 -- IGBT/RConn1

== system svpwm/Motor/Subsystem7/Subsystem5 ==
  Vdn : Inport
  Diode : spsDiodeLib/Diode  Ron=0.001  Lon=0  Vf=0.8  IC=0  UseSnubber=0  Rs=500  Cs=250e-9  Measurements=on
  IGBT : spsIGBTLib/IGBT  Ron=0.001  Lon=0  Vf=1  Tf=1e-6  Tt=2e-6  IC=0  Rs=1e5  Cs=inf  Measurements=on
  Terminator : Terminator
  Terminator1 : Terminator
  up : PMIOPort  Side=Left
  dn : PMIOPort  Port=2  Side=Left
  wires:
  Diode/1 -> Terminator/1
  IGBT/1 -> Terminator1/1
  Vdn/1 -> IGBT/1
  connections:
  IGBT/RConn1 -- Diode/LConn1 -- dn/RConn1
  up/RConn1 -- Diode/RConn1 -- IGBT/LConn1

== system svpwm/Motor/Subsystem7/Subsystem6 ==
  Wdn : Inport
  Diode : spsDiodeLib/Diode  Ron=0.001  Lon=0  Vf=0.8  IC=0  UseSnubber=0  Rs=500  Cs=250e-9  Measurements=on
  IGBT : spsIGBTLib/IGBT  Ron=0.001  Lon=0  Vf=1  Tf=1e-6  Tt=2e-6  IC=0  Rs=1e5  Cs=inf  Measurements=on
  Terminator : Terminator
  Terminator1 : Terminator
  up : PMIOPort  Side=Left
  dn : PMIOPort  Port=2  Side=Left
  wires:
  Wdn/1 -> IGBT/1
  IGBT/1 -> Terminator1/1
  Diode/1 -> Terminator/1
  connections:
  IGBT/LConn1 -- Diode/RConn1 -- up/RConn1
  dn/RConn1 -- Diode/LConn1 -- IGBT/RConn1

== system svpwm/SVPWM/DutyCalc1/If Action Subsystem2 ==
  Tcm1 : Inport
  Tcm2 : Inport  Port=2
  Tcm3 : Inport  Port=3
  Action Port : ActionPort  ActionPortLabel=else
  Duty1 : Outport
  Duty2 : Outport  Port=2
  Duty3 : Outport  Port=3
  wires:
  Tcm1/1 -> Duty1/1
  Tcm2/1 -> Duty2/1
  Tcm3/1 -> Duty3/1

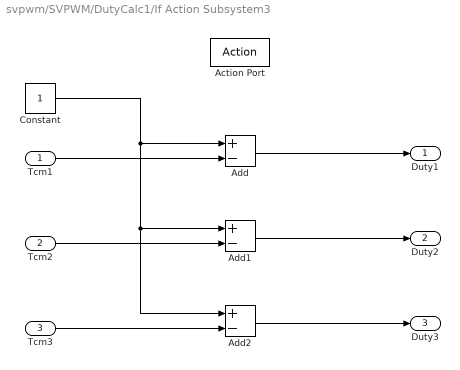
== system svpwm/SVPWM/DutyCalc1/If Action Subsystem3 ==
  Tcm1 : Inport
  Tcm2 : Inport  Port=2
  Tcm3 : Inport  Port=3
  Action Port : ActionPort  ActionPortLabel=if(u1 == 1)
  Add : Sum  Inputs=+-
  Add1 : Sum  Inputs=+-
  Add2 : Sum  Inputs=+-
  Constant : Constant  OutDataTypeStr=Inherit: Inherit via back propagation
  Duty1 : Outport
  Duty2 : Outport  Port=2
  Duty3 : Outport  Port=3
  wires:
  Add2/1 -> Duty3/1
  Add1/1 -> Duty2/1
  Add/1 -> Duty1/1
  Tcm3/1 -> Add2/2
  Tcm2/1 -> Add1/2
  Tcm1/1 -> Add/2
  Constant/1 -> Add/1, Add1/1, Add2/1

== system svpwm/SVPWM/OverModulation/OverModulationCalc ==
  T1 : Inport
  T2 : Inport  Port=2
  Add : Sum
  If : If  IfExpression=u1 > 1
  If Action Subsystem : Subsystem  TreatAsAtomicUnit=on
  If Action Subsystem1 : Subsystem  TreatAsAtomicUnit=on
  Merge : Merge
  Merge1 : Merge
  T1_ : Outport
  T2_ : Outport  Port=2
  wires:
  Merge/1 -> T1_/1
  If/1 -> If Action Subsystem/Action
  If/2 -> If Action Subsystem1/Action
  If Action Subsystem/1(T1_) -> Merge/1
  If Action Subsystem1/1(T1_) -> Merge/2
  If Action Subsystem1/2(T2_) -> Merge1/2
  Merge1/1 -> T2_/1
  If Action Subsystem/2(T2_) -> Merge1/1
  T2/1 -> If Action Subsystem1/2(T2), If Action Subsystem/2(T2), Add/2
  T1/1 -> If Action Subsystem/1(T1), If Action Subsystem1/1(T1), Add/1
  Add/1 -> If Action Subsystem/3(Sum), If/1

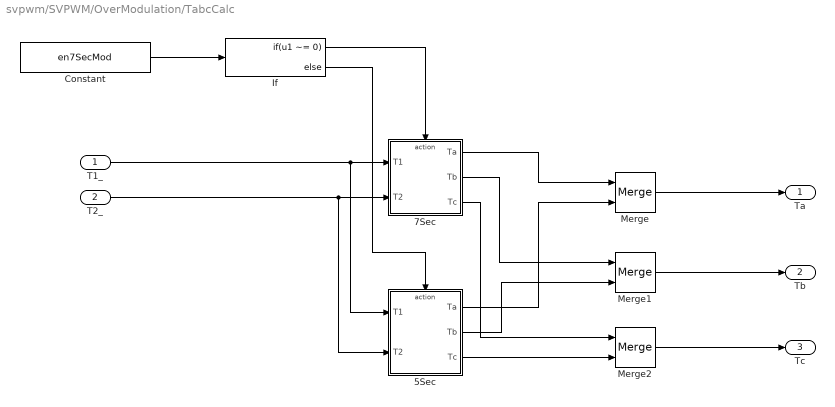
== system svpwm/SVPWM/OverModulation/TabcCalc ==
  T1_ : Inport
  T2_ : Inport  Port=2
  5Sec : Subsystem  TreatAsAtomicUnit=on
  7Sec : Subsystem  TreatAsAtomicUnit=on
  Constant : Constant  Value=en7SecMod
  If : If  IfExpression=u1 ~= 0
  Merge : Merge
  Merge1 : Merge
  Merge2 : Merge
  Ta : Outport
  Tb : Outport  Port=2
  Tc : Outport  Port=3
  wires:
  Constant/1 -> If/1
  If/1 -> 7Sec/Action
  If/2 -> 5Sec/Action
  T1_/1 -> 5Sec/1(T1), 7Sec/1(T1)
  T2_/1 -> 5Sec/2(T2), 7Sec/2(T2)
  Merge/1 -> Ta/1
  7Sec/1(Ta) -> Merge/1
  5Sec/1(Ta) -> Merge/2
  Merge1/1 -> Tb/1
  Merge2/1 -> Tc/1
  7Sec/2(Tb) -> Merge1/1
  5Sec/2(Tb) -> Merge1/2
  7Sec/3(Tc) -> Merge2/1
  5Sec/3(Tc) -> Merge2/2

== system svpwm/SVPWM/OverModulation/OverModulationCalc/If Action Subsystem ==
  T1 : Inport
  T2 : Inport  Port=2
  Sum : Inport  Port=3
  Action Port : ActionPort  ActionPortLabel=if(u1 > 1)
  Divide : Product  Inputs=*/
  Divide1 : Product  Inputs=*/
  T1_ : Outport
  T2_ : Outport  Port=2
  wires:
  T1/1 -> Divide/1
  T2/1 -> Divide1/1
  Sum/1 -> Divide/2, Divide1/2
  Divide/1 -> T1_/1
  Divide1/1 -> T2_/1

== system svpwm/SVPWM/OverModulation/OverModulationCalc/If Action Subsystem1 ==
  T1 : Inport
  T2 : Inport  Port=2
  Action Port : ActionPort  ActionPortLabel=else
  T1_ : Outport
  T2_ : Outport  Port=2
  wires:
  T1/1 -> T1_/1
  T2/1 -> T2_/1

== system svpwm/SVPWM/OverModulation/TabcCalc/5Sec ==
  note: 零矢量选择全部为U7(1,1,1)
  T1 : Inport
  T2 : Inport  Port=2
  Action Port : ActionPort  ActionPortLabel=else
  Add2 : Sum
  Constant : Constant  Value=0  OutDataTypeStr=single
  Ta : Outport
  Tb : Outport  Port=2
  Tc : Outport  Port=3
  wires:
  Add2/1 -> Tc/1
  T2/1 -> Tb/1, Add2/1
  T1/1 -> Add2/2
  Constant/1 -> Ta/1

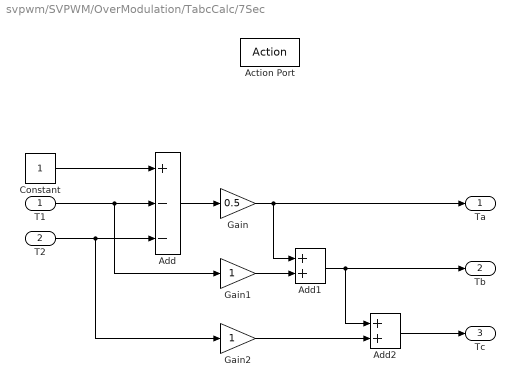
== system svpwm/SVPWM/OverModulation/TabcCalc/7Sec ==
  T1 : Inport
  T2 : Inport  Port=2
  Action Port : ActionPort  ActionPortLabel=if(u1 ~= 0)
  Add : Sum  Inputs=+--
  Add1 : Sum
  Add2 : Sum
  Constant : Constant  OutDataTypeStr=single
  Gain : Gain  Gain=0.5
  Gain1 : Gain
  Gain2 : Gain
  Ta : Outport
  Tb : Outport  Port=2
  Tc : Outport  Port=3
  wires:
  Constant/1 -> Add/1
  T1/1 -> Gain1/1, Add/2
  T2/1 -> Gain2/1, Add/3
  Add/1 -> Gain/1
  Gain/1 -> Add1/1, Ta/1
  Add1/1 -> Add2/1, Tb/1
  Gain1/1 -> Add1/2
  Gain2/1 -> Add2/2
  Add2/1 -> Tc/1
